simulink model "Lcontainer_simNN"  (R2018b)
settings: Solver=FixedStepAuto  StartTime=0.0  StopTime=50  FixedStep=0.1  RelTol=1e-3
libraries: neural x548, simulink x2
(part 2 of 26)

== system Lcontainer_simNN/Lcontainer Plant/NN Plant2 LContainer /Layer 2 ==
  "a{1} " : Inport  PortDimensions=100
      mask Display: e = 0.06;c1 = [120 230 180]/255;c2 = ([120 230 180]+0)/(256+128);c3 = ([120 230 180]+128)/(256+128);patch([0 1 1 0],[0 0 1 1],c1);patch([0 1 1 1-e 1-e 0+e],[0 0 1 1-e 0+e 0+e],c2);patch([0 0 1 1-e 0+e 0+e],[0 1 1 1-e 1-e 0+e],c3);plot([0 1 1 0 0],[0 0 1 1 0]);
  Delays 1 : Subsystem
      mask Display: e = 0.06;c1 = [120 150 230]/255;c2 = ([120 150 230]+0)/383;c3 = ([120 150 230]+128)/383;patch([0 1 1 0],[0 0 1 1],c1);patch([0 1 1 1-e 1-e 0+e],[0 0 1 1-e 0+e 0+e],c2);patch([0 0 1 1-e 0+e 0+e],[0 1 1 1-e 1-e 0+e],c3);plot([0 1 1 0 0],[0 0 1 1 0]);disp('0');
  "LW{2,1}" : Subsystem
      mask Display: e = 0.06;c1 = [120 150 230]/255;c2 = ([120 150 230]+0)/383;c3 = ([120 150 230]+128)/383;patch([0 1 1 0],[0 0 1 1],c1);patch([0 1 1 1-e 1-e 0+e],[0 0 1 1-e 0+e 0+e],c2);patch([0 0 1 1-e 0+e 0+e],[0 1 1 1-e 1-e 0+e],c3);plot([0 1 1 0 0],[0 0 1 1 0]);disp('W');
  "b{2}" : Constant  Value=[1.457948400383569431681962669244967401027679443359375;-1.4363642103566884866694408628973178565502166748046875;-1.406748453442117519074372467002831399440765380859375;1.394290982335961270877078277408145368099212646484375;1.343050602780088365051369692082516849040985107421875;-1.3179011826984050603783771293819881975650787353515625;-1.28828542578383409278330873348750174045562744140625;-1.2586696688692631251882403375930152833461761474609375;1.2223852652341660185442151487222872674465179443359375;-1.1994381550401211899981035458040423691272735595703125;-1.1698223981255504444476400749408639967441558837890625;-1.1402066412109796988971766040776856243610382080078125;-1.1105908842964087313021082081831991672515869140625;-1.0809751273818377637070398122887127101421356201171875;1.0433017757962634863844186838832683861255645751953125;-1.021743613552696050561507945531047880649566650390625;-0.99212785663812497194413708712090738117694854736328125;0.974947622331601149170410280930809676647186279296875;0.93923084963295500049440533985034562647342681884765625;0.89712165434562074484148297415231354534626007080078125;-0.87366482897984154565307335360557772219181060791015625;-0.8440490720652704670357024951954372227191925048828125;-0.8144333151506997214852390243322588503360748291015625;0.76410477772533036411317652891739271581172943115234375;0.75393318687811305967017005968955345451831817626953125;-0.72558604440698692972233629916445352137088775634765625;-0.695970287492416073149570365785621106624603271484375;-0.69089749486050655580271495637134648859500885009765625;0.64175029841416109110951992988702841103076934814453125;-0.61638215668072804387378482715575955808162689208984375;-0.57750725983413253583620416975463740527629852294921875;-0.54789150291956156824113577386015094816684722900390625;0.54725443631476811123803827285883016884326934814453125;0.519349916881416628910983490641228854656219482421875;-0.459044232175848943011686742465826682746410369873046875;0.471514947786536298135473543879925273358821868896484375;0.393658022045692279622386422488489188253879547119140625;0.398286745112922890843520917769637890160083770751953125;-0.340581204517565405698320546434842981398105621337890625;-0.273673197686332081435267582492087967693805694580078125;-0.28134969068842352601933498590369708836078643798828125;-0.2525958777538104271798147237859666347503662109375;0.217389693880161438688247699246858246624469757080078125;-0.1809853591225712710066630961591727100312709808349609375;0.2203228374720167803690884511524927802383899688720703125;-0.1714219562968098131694461017104913480579853057861328125;-0.1667076294070486131015940145516651682555675506591796875;0.1378102788899506492281687997092376463115215301513671875;-0.0325044531091032984360111868227249942719936370849609375;0.00757822062037809794643461458463207236491143703460693359375;0.0698805671416244944538220806862227618694305419921875;-0.044423635371856305675830611789933755062520503997802734375;-0.06213672982577456149755334990913979709148406982421875;0.1685070351320023807062398191192187368869781494140625;0.1419476914833218972322725903723039664328098297119140625;-0.1628866630301400164615444055016268976032733917236328125;0.1976434507178117805370476389725808985531330108642578125;0.2212012222569459118926005203320528380572795867919921875;0.2399253354382317182658113097204477526247501373291015625;0.2611323764452924134360500829643569886684417724609375;-0.31096544760299449361440338179818354547023773193359375;-0.34058120451756523916486685266136191785335540771484375;-0.3701969614321363177822377110715024173259735107421875;0.399113453267117612721648356455261819064617156982421875;-0.429428475261278197461223271602648310363292694091796875;-0.459044232175848943011686742465826682746410369873046875;-0.488659989090419688562150213329005055129528045654296875;-0.51827574600499082269067230299697257578372955322265625;0.595636561711085921189123837393708527088165283203125;-0.57750725983413264685850663227029144763946533203125 ...(+1636 chars)]
      mask Display: e = 0.06;c1 = [120 150 230]/255;c2 = ([120 150 230]+0)/383;c3 = ([120 150 230]+128)/383;patch([0 1 1 0],[0 0 1 1],c1);patch([0 1 1 1-e 1-e 0+e],[0 0 1 1-e 0+e 0+e],c2);patch([0 0 1 1-e 0+e 0+e],[0 1 1 1-e 1-e 0+e],c3);plot([0 1 1 0 0],[0 0 1 1 0]);disp('b');
  netsum : Sum  Inputs=2  SaturateOnIntegerOverflow=on  InputSameDT=on  OutDataTypeStr=Inherit: Same as first input
      mask Display: e = 0.06;c1 = [120 150 230]/255;c2 = ([120 150 230]+0)/383;c3 = ([120 150 230]+128)/383;patch([0 1 1 0],[0 0 1 1],c1);patch([0 1 1 1-e 1-e 0+e],[0 0 1 1-e 0+e 0+e],c2);patch([0 0 1 1-e 0+e 0+e],[0 1 1 1-e 1-e 0+e],c3);plot([0 1 1 0 0],[0 0 1 1 0]);disp('+');
  poslin : neural/Transfer Functions/poslin
      settings: SourceProductName=Neural Network Toolbox  SourceProductBaseCode=NN
  "a{2}" : Outport  InitialOutput=[0;0;0;0;0;0;0;0;0;0;0;0;0;0;0;0;0;0;0;0;0;0;0;0;0;0;0;0;0;0;0;0;0;0;0;0;0;0;0;0;0;0;0;0;0;0;0;0;0;0;0;0;0;0;0;0;0;0;0;0;0;0;0;0;0;0;0;0;0;0;0;0;0;0;0;0;0;0;0;0;0;0;0;0;0;0;0;0;0;0;0;0;0;0;0;0;0;0;0;0]
      mask Display: e = 0.06;c1 = [120 230 180]/255;c2 = ([120 230 180]+0)/(256+128);c3 = ([120 230 180]+128)/(256+128);patch([0 1 1 0],[0 0 1 1],c1);patch([0 1 1 1-e 1-e 0+e],[0 0 1 1-e 0+e 0+e],c2);patch([0 0 1 1-e 0+e 0+e],[0 1 1 1-e 1-e 0+e],c3);plot([0 1 1 0 0],[0 0 1 1 0]);
  wires:
  poslin/1 -> "a{2}"/1
  netsum/1 -> poslin/1
  "b{2}"/1 -> netsum/2
  "LW{2,1}"/1("lz{2,1}") -> netsum/1
  Delays 1/1("pd{2,1}") -> "LW{2,1}"/1("ad{2,1}")
  "a{1} "/1 -> Delays 1/1("p{2}")

== system Lcontainer_simNN/Lcontainer Plant/NN Plant2 LContainer /Layer 3 ==
  "a{2} " : Inport  PortDimensions=100
      mask Display: e = 0.06;c1 = [120 230 180]/255;c2 = ([120 230 180]+0)/(256+128);c3 = ([120 230 180]+128)/(256+128);patch([0 1 1 0],[0 0 1 1],c1);patch([0 1 1 1-e 1-e 0+e],[0 0 1 1-e 0+e 0+e],c2);patch([0 0 1 1-e 0+e 0+e],[0 1 1 1-e 1-e 0+e],c3);plot([0 1 1 0 0],[0 0 1 1 0]);
  Delays 1 : Subsystem
      mask Display: e = 0.06;c1 = [120 150 230]/255;c2 = ([120 150 230]+0)/383;c3 = ([120 150 230]+128)/383;patch([0 1 1 0],[0 0 1 1],c1);patch([0 1 1 1-e 1-e 0+e],[0 0 1 1-e 0+e 0+e],c2);patch([0 0 1 1-e 0+e 0+e],[0 1 1 1-e 1-e 0+e],c3);plot([0 1 1 0 0],[0 0 1 1 0]);disp('0');
  "LW{3,2}" : Subsystem
      mask Display: e = 0.06;c1 = [120 150 230]/255;c2 = ([120 150 230]+0)/383;c3 = ([120 150 230]+128)/383;patch([0 1 1 0],[0 0 1 1],c1);patch([0 1 1 1-e 1-e 0+e],[0 0 1 1-e 0+e 0+e],c2);patch([0 0 1 1-e 0+e 0+e],[0 1 1 1-e 1-e 0+e],c3);plot([0 1 1 0 0],[0 0 1 1 0]);disp('W');
  "b{3}" : Constant  Value=[-1.46597996727125945426450925879180431365966796875;1.4380972050561606767615785429370589554309844970703125;-1.4094507077230693514735548887983895838260650634765625;1.377132696527546773523908996139653027057647705078125;-1.3475169396129758059288406002451665699481964111328125;1.3222205102540665055954605122678913176059722900390625;1.287261723765149579179478678270243108272552490234375;-1.2586696688692631251882403375930152833461761474609375;-1.214413550208770953275916326674632728099822998046875;1.207705732345353499823659149114973843097686767578125;1.170906844241318633947912530857138335704803466796875;1.14052278062657297397208822076208889484405517578125;-1.1105908842964087313021082081831991672515869140625;-1.0809751273818377637070398122887127101421356201171875;-1.051359370467266796111971416394226253032684326171875;1.0345398482620768998430094143259339034557342529296875;0.98462868392107771864374399228836409747600555419921875;-0.96251209972355422639367361625772900879383087158203125;-0.93289634280898325879860522036324255168437957763671875;-0.9032805858944124022258392869844101369380950927734375;0.87361531872434772250102241741842590272426605224609375;0.84918309653226697886196916442713700234889984130859375;-0.82422358600135492423532923567108809947967529296875;0.7981335850852939728383717010729014873504638671875;-0.75520180132155789731740469505893997848033905029296875;-0.71266608364973171862999379300163127481937408447265625;0.7031181572743301355643552597030065953731536865234375;0.6644480673862684927399868684005923569202423095703125;0.62934049865035424087267301729298196732997894287109375;0.60034368662445014575013146895798854529857635498046875;-0.5774463190394214517908721973071806132793426513671875;0.53065504118274497979967918581678532063961029052734375;-0.5196572917370030353367837960831820964813232421875;0.48865998909041985509560390710248611867427825927734375;0.455103207608760940150460783115704543888568878173828125;-0.43272782351088789898341246953350491821765899658203125;0.40101910254801265143242972044390626251697540283203125;-0.370196961432136151248784017298021353781223297119140625;-0.340581204517565405698320546434842981398105621337890625;0.30573008773446519459326964351930655539035797119140625;-0.29946517875288491961072168123791925609111785888671875;0.244922075093180591220942687868955545127391815185546875;0.2221181768592817018515006566303782165050506591796875;-0.1925024199447107620120078763648052699863910675048828125;-0.1590180409209177303520021951044327579438686370849609375;0.12491579110304018573884832221665419638156890869140625;0.10365514920099816453813446059939451515674591064453125;0.07403939228642723857642948814827832393348217010498046875;0.055164255290131525288899183578905649483203887939453125;-0.00695933394758176636363256051254211342893540859222412109375;-0.0038791936118102369850102473236574951442889869213104248046875;-0.048093045723783756084657170504215173423290252685546875;0.07406245336093873754546024201772524975240230560302734375;0.114902335864814519883481125361868180334568023681640625;0.13327090611556891008859793146257288753986358642578125;0.1512286677702585624416542486869730055332183837890625;0.1925024199447107620120078763648052699863910675048828125;0.2272188462606656578213204511484946124255657196044921875;-0.24961375829947696214361485544941388070583343505859375;-0.290323978755354261682697369906236417591571807861328125;-0.31096544760299449361440338179818354547023773193359375;0.34463016884257668959179454759578220546245574951171875;-0.3701969614321363177822377110715024173259735107421875;0.40793759485472402825934068459901027381420135498046875;-0.427514028800229206606076104435487650334835052490234375;-0.459044232175848943011686742465826682746410369873046875;-0.486218613453763104370608516546781174838542938232421875;0.52899111212253779878977866246714256703853607177734375;-0.5530564283990491158959912354475818574428558349609375;0.56916360397631271528240404222742654383182525634765625;-0.6038466478129758119308689856552518904209136962890625 ...(+1582 chars)]
      mask Display: e = 0.06;c1 = [120 150 230]/255;c2 = ([120 150 230]+0)/383;c3 = ([120 150 230]+128)/383;patch([0 1 1 0],[0 0 1 1],c1);patch([0 1 1 1-e 1-e 0+e],[0 0 1 1-e 0+e 0+e],c2);patch([0 0 1 1-e 0+e 0+e],[0 1 1 1-e 1-e 0+e],c3);plot([0 1 1 0 0],[0 0 1 1 0]);disp('b');
  netsum : Sum  Inputs=2  SaturateOnIntegerOverflow=on  InputSameDT=on  OutDataTypeStr=Inherit: Same as first input
      mask Display: e = 0.06;c1 = [120 150 230]/255;c2 = ([120 150 230]+0)/383;c3 = ([120 150 230]+128)/383;patch([0 1 1 0],[0 0 1 1],c1);patch([0 1 1 1-e 1-e 0+e],[0 0 1 1-e 0+e 0+e],c2);patch([0 0 1 1-e 0+e 0+e],[0 1 1 1-e 1-e 0+e],c3);plot([0 1 1 0 0],[0 0 1 1 0]);disp('+');
  poslin : neural/Transfer Functions/poslin
      settings: SourceProductName=Neural Network Toolbox  SourceProductBaseCode=NN
  "a{3}" : Outport  InitialOutput=[0;0;0;0;0;0;0;0;0;0;0;0;0;0;0;0;0;0;0;0;0;0;0;0;0;0;0;0;0;0;0;0;0;0;0;0;0;0;0;0;0;0;0;0;0;0;0;0;0;0;0;0;0;0;0;0;0;0;0;0;0;0;0;0;0;0;0;0;0;0;0;0;0;0;0;0;0;0;0;0;0;0;0;0;0;0;0;0;0;0;0;0;0;0;0;0;0;0;0;0]
      mask Display: e = 0.06;c1 = [120 230 180]/255;c2 = ([120 230 180]+0)/(256+128);c3 = ([120 230 180]+128)/(256+128);patch([0 1 1 0],[0 0 1 1],c1);patch([0 1 1 1-e 1-e 0+e],[0 0 1 1-e 0+e 0+e],c2);patch([0 0 1 1-e 0+e 0+e],[0 1 1 1-e 1-e 0+e],c3);plot([0 1 1 0 0],[0 0 1 1 0]);
  wires:
  poslin/1 -> "a{3}"/1
  netsum/1 -> poslin/1
  "b{3}"/1 -> netsum/2
  "LW{3,2}"/1("lz{3,2}") -> netsum/1
  Delays 1/1("pd{3,2}") -> "LW{3,2}"/1("ad{3,2}")
  "a{2} "/1 -> Delays 1/1("p{3}")

== system Lcontainer_simNN/Lcontainer Plant/NN Plant2 LContainer /Layer 4 ==
  "a{3} " : Inport  PortDimensions=100
      mask Display: e = 0.06;c1 = [120 230 180]/255;c2 = ([120 230 180]+0)/(256+128);c3 = ([120 230 180]+128)/(256+128);patch([0 1 1 0],[0 0 1 1],c1);patch([0 1 1 1-e 1-e 0+e],[0 0 1 1-e 0+e 0+e],c2);patch([0 0 1 1-e 0+e 0+e],[0 1 1 1-e 1-e 0+e],c3);plot([0 1 1 0 0],[0 0 1 1 0]);
  Delays 1 : Subsystem
      mask Display: e = 0.06;c1 = [120 150 230]/255;c2 = ([120 150 230]+0)/383;c3 = ([120 150 230]+128)/383;patch([0 1 1 0],[0 0 1 1],c1);patch([0 1 1 1-e 1-e 0+e],[0 0 1 1-e 0+e 0+e],c2);patch([0 0 1 1-e 0+e 0+e],[0 1 1 1-e 1-e 0+e],c3);plot([0 1 1 0 0],[0 0 1 1 0]);disp('0');
  "LW{4,3}" : Subsystem
      mask Display: e = 0.06;c1 = [120 150 230]/255;c2 = ([120 150 230]+0)/383;c3 = ([120 150 230]+128)/383;patch([0 1 1 0],[0 0 1 1],c1);patch([0 1 1 1-e 1-e 0+e],[0 0 1 1-e 0+e 0+e],c2);patch([0 0 1 1-e 0+e 0+e],[0 1 1 1-e 1-e 0+e],c3);plot([0 1 1 0 0],[0 0 1 1 0]);disp('W');
  "b{4}" : Constant  Value=[1.475031812836384847997805991326458752155303955078125;-1.4363642103566884866694408628973178565502166748046875;1.4052526132200060526855622811126522719860076904296875;1.3778405019348618498753467065398581326007843017578125;1.348269422195949029941175467683933675289154052734375;1.327242193372675682638828220660798251628875732421875;1.2842240181857615954896800758433528244495391845703125;-1.2586696688692631251882403375930152833461761474609375;-1.229053911954692157593171941698528826236724853515625;1.2014513944001052880850011206348426640033721923828125;-1.1698223981255504444476400749408639967441558837890625;1.1376373558437820054933808933128602802753448486328125;-1.10203380461833599923693327582441270351409912109375;-1.0809751273818377637070398122887127101421356201171875;1.062561570020715606688099796883761882781982421875;1.01475098891088411079408615478314459323883056640625;0.9941107130229946964306009249412454664707183837890625;0.96321123894414839572419850810547359287738800048828125;-0.93289634280898325879860522036324255168437957763671875;-0.9032805858944124022258392869844101369380950927734375;0.87020229472582399932178987000952474772930145263671875;-0.8440490720652704670357024951954372227191925048828125;-0.8144333151506997214852390243322588503360748291015625;0.77852515049172887895423400550498627126216888427734375;0.7655048799950510129974645678885281085968017578125;0.72558604440698692972233629916445352137088775634765625;0.6957384199568921179235303497989661991596221923828125;-0.66635453057784521657680443240678869187831878662109375;-0.6367387736632743600040384990279562771320343017578125;-0.6071230167487033924089701031334698200225830078125;-0.5776078867769613989224808392464183270931243896484375;0.54638319083786368590693882651976309716701507568359375;0.51803568781976572221736887513543479144573211669921875;0.4890230513130762179940802525379694998264312744140625;-0.459044232175848943011686742465826682746410369873046875;0.43022274283388128868210742439259774982929229736328125;0.400799602124944864822708723295363597571849822998046875;-0.370196961432136151248784017298021353781223297119140625;-0.340581204517565405698320546434842981398105621337890625;0.31039785334973324371077296746079809963703155517578125;0.28134969068842352601933498590369708836078643798828125;0.25573396074734910943249133197241462767124176025390625;-0.2221181768592817018515006566303782165050506591796875;0.1959819103893961356188668787581264041364192962646484375;-0.1628866630301400164615444055016268976032733917236328125;-0.133270906115569076622051625236053951084613800048828125;-0.10322093476565498415542521115639829076826572418212890625;0.0740172856772971510253000815282575786113739013671875;-0.03637773195881842391852245555128320120275020599365234375;0.0151923328766308575465959762595957727171480655670166015625;0.00123844623489508995871355434559291097684763371944427490234375;0.044342673372869602366197483434007153846323490142822265625;-0.0713051780206427066044483353834948502480983734130859375;0.10381438511427398818653955459012649953365325927734375;0.1329033682704214569536560475171427242457866668701171875;-0.1628866630301400164615444055016268976032733917236328125;0.20287394113381640448068310433882288634777069091796875;-0.224739801778688630395919290094752795994281768798828125;-0.2523140276705415629976414493285119533538818359375;0.278967676165778666330652413307689130306243896484375;0.31096544760299449361440338179818354547023773193359375;-0.34058120451756523916486685266136191785335540771484375;-0.3701969614321363177822377110715024173259735107421875;0.422833268995362610009891568552120588719844818115234375;-0.429428475261278197461223271602648310363292694091796875;-0.459044232175848943011686742465826682746410369873046875;0.488659989090419688562150213329005055129528045654296875;-0.51827574600499082269067230299697257578372955322265625;-0.54789150291956156824113577386015094816684722900390625;-0.5815063350459450663976213036221452057361602783203125;-0.6071230167487033924089701031334698200225830078125 ...(+1596 chars)]
      mask Display: e = 0.06;c1 = [120 150 230]/255;c2 = ([120 150 230]+0)/383;c3 = ([120 150 230]+128)/383;patch([0 1 1 0],[0 0 1 1],c1);patch([0 1 1 1-e 1-e 0+e],[0 0 1 1-e 0+e 0+e],c2);patch([0 0 1 1-e 0+e 0+e],[0 1 1 1-e 1-e 0+e],c3);plot([0 1 1 0 0],[0 0 1 1 0]);disp('b');
  netsum : Sum  Inputs=2  SaturateOnIntegerOverflow=on  InputSameDT=on  OutDataTypeStr=Inherit: Same as first input
      mask Display: e = 0.06;c1 = [120 150 230]/255;c2 = ([120 150 230]+0)/383;c3 = ([120 150 230]+128)/383;patch([0 1 1 0],[0 0 1 1],c1);patch([0 1 1 1-e 1-e 0+e],[0 0 1 1-e 0+e 0+e],c2);patch([0 0 1 1-e 0+e 0+e],[0 1 1 1-e 1-e 0+e],c3);plot([0 1 1 0 0],[0 0 1 1 0]);disp('+');
  poslin : neural/Transfer Functions/poslin
      settings: SourceProductName=Neural Network Toolbox  SourceProductBaseCode=NN
  "a{4}" : Outport  InitialOutput=[0;0;0;0;0;0;0;0;0;0;0;0;0;0;0;0;0;0;0;0;0;0;0;0;0;0;0;0;0;0;0;0;0;0;0;0;0;0;0;0;0;0;0;0;0;0;0;0;0;0;0;0;0;0;0;0;0;0;0;0;0;0;0;0;0;0;0;0;0;0;0;0;0;0;0;0;0;0;0;0;0;0;0;0;0;0;0;0;0;0;0;0;0;0;0;0;0;0;0;0]
      mask Display: e = 0.06;c1 = [120 230 180]/255;c2 = ([120 230 180]+0)/(256+128);c3 = ([120 230 180]+128)/(256+128);patch([0 1 1 0],[0 0 1 1],c1);patch([0 1 1 1-e 1-e 0+e],[0 0 1 1-e 0+e 0+e],c2);patch([0 0 1 1-e 0+e 0+e],[0 1 1 1-e 1-e 0+e],c3);plot([0 1 1 0 0],[0 0 1 1 0]);
  wires:
  poslin/1 -> "a{4}"/1
  netsum/1 -> poslin/1
  "b{4}"/1 -> netsum/2
  "LW{4,3}"/1("lz{4,3}") -> netsum/1
  Delays 1/1("pd{4,3}") -> "LW{4,3}"/1("ad{4,3}")
  "a{3} "/1 -> Delays 1/1("p{4}")

== system Lcontainer_simNN/Lcontainer Plant/NN Plant2 LContainer /Layer 5 ==
  "a{4} " : Inport  PortDimensions=100
      mask Display: e = 0.06;c1 = [120 230 180]/255;c2 = ([120 230 180]+0)/(256+128);c3 = ([120 230 180]+128)/(256+128);patch([0 1 1 0],[0 0 1 1],c1);patch([0 1 1 1-e 1-e 0+e],[0 0 1 1-e 0+e 0+e],c2);patch([0 0 1 1-e 0+e 0+e],[0 1 1 1-e 1-e 0+e],c3);plot([0 1 1 0 0],[0 0 1 1 0]);
  Delays 1 : Subsystem
      mask Display: e = 0.06;c1 = [120 150 230]/255;c2 = ([120 150 230]+0)/383;c3 = ([120 150 230]+128)/383;patch([0 1 1 0],[0 0 1 1],c1);patch([0 1 1 1-e 1-e 0+e],[0 0 1 1-e 0+e 0+e],c2);patch([0 0 1 1-e 0+e 0+e],[0 1 1 1-e 1-e 0+e],c3);plot([0 1 1 0 0],[0 0 1 1 0]);disp('0');
  "LW{5,4}" : Subsystem
      mask Display: e = 0.06;c1 = [120 150 230]/255;c2 = ([120 150 230]+0)/383;c3 = ([120 150 230]+128)/383;patch([0 1 1 0],[0 0 1 1],c1);patch([0 1 1 1-e 1-e 0+e],[0 0 1 1-e 0+e 0+e],c2);patch([0 0 1 1-e 0+e 0+e],[0 1 1 1-e 1-e 0+e],c3);plot([0 1 1 0 0],[0 0 1 1 0]);disp('W');
  "b{5}" : Constant  Value=[0;0.0136255313037318658009322547286501503549516201019287109375;-0.01425084325618868920371173913963502855040132999420166015625;0.0372185869617984443902258817615802399814128875732421875;-0.000208133641306395785787464181026962251053191721439361572265625;-0.031520961552764910351687177580970455892384052276611328125;0.0064930429514983116490167702750113676302134990692138671875;-0.01204129612258644614619651491693730349652469158172607421875;0.006255900979858426171065222121114857145585119724273681640625]
      mask Display: e = 0.06;c1 = [120 150 230]/255;c2 = ([120 150 230]+0)/383;c3 = ([120 150 230]+128)/383;patch([0 1 1 0],[0 0 1 1],c1);patch([0 1 1 1-e 1-e 0+e],[0 0 1 1-e 0+e 0+e],c2);patch([0 0 1 1-e 0+e 0+e],[0 1 1 1-e 1-e 0+e],c3);plot([0 1 1 0 0],[0 0 1 1 0]);disp('b');
  netsum : Sum  Inputs=2  SaturateOnIntegerOverflow=on  InputSameDT=on  OutDataTypeStr=Inherit: Same as first input
      mask Display: e = 0.06;c1 = [120 150 230]/255;c2 = ([120 150 230]+0)/383;c3 = ([120 150 230]+128)/383;patch([0 1 1 0],[0 0 1 1],c1);patch([0 1 1 1-e 1-e 0+e],[0 0 1 1-e 0+e 0+e],c2);patch([0 0 1 1-e 0+e 0+e],[0 1 1 1-e 1-e 0+e],c3);plot([0 1 1 0 0],[0 0 1 1 0]);disp('+');
  purelin : neural/Transfer Functions/purelin
  "a{5}" : Outport  InitialOutput=[0;0;0;0;0;0;0;0;0]
      mask Display: e = 0.06;c1 = [120 230 180]/255;c2 = ([120 230 180]+0)/(256+128);c3 = ([120 230 180]+128)/(256+128);patch([0 1 1 0],[0 0 1 1],c1);patch([0 1 1 1-e 1-e 0+e],[0 0 1 1-e 0+e 0+e],c2);patch([0 0 1 1-e 0+e 0+e],[0 1 1 1-e 1-e 0+e],c3);plot([0 1 1 0 0],[0 0 1 1 0]);
  wires:
  purelin/1 -> "a{5}"/1
  netsum/1 -> purelin/1
  "b{5}"/1 -> netsum/2
  "LW{5,4}"/1("lz{5,4}") -> netsum/1
  Delays 1/1("pd{5,4}") -> "LW{5,4}"/1("ad{5,4}")
  "a{4} "/1 -> Delays 1/1("p{5}")

== system Lcontainer_simNN/Lcontainer Plant/NN Plant2 LContainer /Process Input 1 ==
  x : Inport  PortDimensions=10
      mask Display: e = 0.06;c1 = [120 230 180]/255;c2 = ([120 230 180]+0)/(256+128);c3 = ([120 230 180]+128)/(256+128);patch([0 1 1 0],[0 0 1 1],c1);patch([0 1 1 1-e 1-e 0+e],[0 0 1 1-e 0+e 0+e],c2);patch([0 0 1 1-e 0+e 0+e],[0 1 1 1-e 1-e 0+e],c3);plot([0 1 1 0 0],[0 0 1 1 0]);
  p : Outport  PortDimensions=10
      mask Display: e = 0.06;c1 = [120 230 180]/255;c2 = ([120 230 180]+0)/(256+128);c3 = ([120 230 180]+128)/(256+128);patch([0 1 1 0],[0 0 1 1],c1);patch([0 1 1 1-e 1-e 0+e],[0 0 1 1-e 0+e 0+e],c2);patch([0 0 1 1-e 0+e 0+e],[0 1 1 1-e 1-e 0+e],c3);plot([0 1 1 0 0],[0 0 1 1 0]);
  wires:
  x/1 -> p/1

== system Lcontainer_simNN/Lcontainer Plant/NN Plant2 LContainer /Process Output 1 ==
  a : Inport  PortDimensions=9
      mask Display: e = 0.06;c1 = [120 230 180]/255;c2 = ([120 230 180]+0)/(256+128);c3 = ([120 230 180]+128)/(256+128);patch([0 1 1 0],[0 0 1 1],c1);patch([0 1 1 1-e 1-e 0+e],[0 0 1 1-e 0+e 0+e],c2);patch([0 0 1 1-e 0+e 0+e],[0 1 1 1-e 1-e 0+e],c3);plot([0 1 1 0 0],[0 0 1 1 0]);
  y : Outport  PortDimensions=9
      mask Display: e = 0.06;c1 = [120 230 180]/255;c2 = ([120 230 180]+0)/(256+128);c3 = ([120 230 180]+128)/(256+128);patch([0 1 1 0],[0 0 1 1],c1);patch([0 1 1 1-e 1-e 0+e],[0 0 1 1-e 0+e 0+e],c2);patch([0 0 1 1-e 0+e 0+e],[0 1 1 1-e 1-e 0+e],c3);plot([0 1 1 0 0],[0 0 1 1 0]);
  wires:
  a/1 -> y/1

== system Lcontainer_simNN/Lcontainer Plant/NN Plant LContainer/Layer 1/Delays 1 ==
  "p{1}" : Inport  PortDimensions=10
      mask Display: e = 0.06;c1 = [120 230 180]/255;c2 = ([120 230 180]+0)/(256+128);c3 = ([120 230 180]+128)/(256+128);patch([0 1 1 0],[0 0 1 1],c1);patch([0 1 1 1-e 1-e 0+e],[0 0 1 1-e 0+e 0+e],c2);patch([0 0 1 1-e 0+e 0+e],[0 1 1 1-e 1-e 0+e],c3);plot([0 1 1 0 0],[0 0 1 1 0]);
  mux : Mux  Inputs=1
      mask Display: e = 0.06;c1 = [120 150 230]/255;c2 = ([120 150 230]+0)/383;c3 = ([120 150 230]+128)/383;patch([0 1 1 0],[0 0 1 1],c1);patch([0 1 1 1-e 1-e 0+e],[0 0 1 1-e 0+e 0+e],c2);patch([0 0 1 1-e 0+e 0+e],[0 1 1 1-e 1-e 0+e],c3);plot([0 1 1 0 0],[0 0 1 1 0]);disp('Mux')
  "pd{1,1}" : Outport
      mask Display: e = 0.06;c1 = [120 230 180]/255;c2 = ([120 230 180]+0)/(256+128);c3 = ([120 230 180]+128)/(256+128);patch([0 1 1 0],[0 0 1 1],c1);patch([0 1 1 1-e 1-e 0+e],[0 0 1 1-e 0+e 0+e],c2);patch([0 0 1 1-e 0+e 0+e],[0 1 1 1-e 1-e 0+e],c3);plot([0 1 1 0 0],[0 0 1 1 0]);
  wires:
  mux/1 -> "pd{1,1}"/1
  "p{1}"/1 -> mux/1
